simulink model "Lab3_1"  (R2021b)
settings: Solver=VariableStepAuto  StartTime=0.0  StopTime=10.0  RelTol=1e-3
libraries: fl_lib x7, nesl_utility x7, ee_lib x6, eeRmsMeasurement x5
settings Model: Creator=coolk  LastModifiedBy=coolk

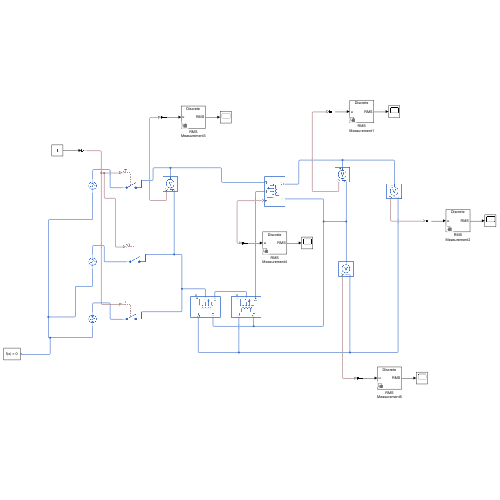
[thumbnail: Simulink's stored preview of the top-level diagram]
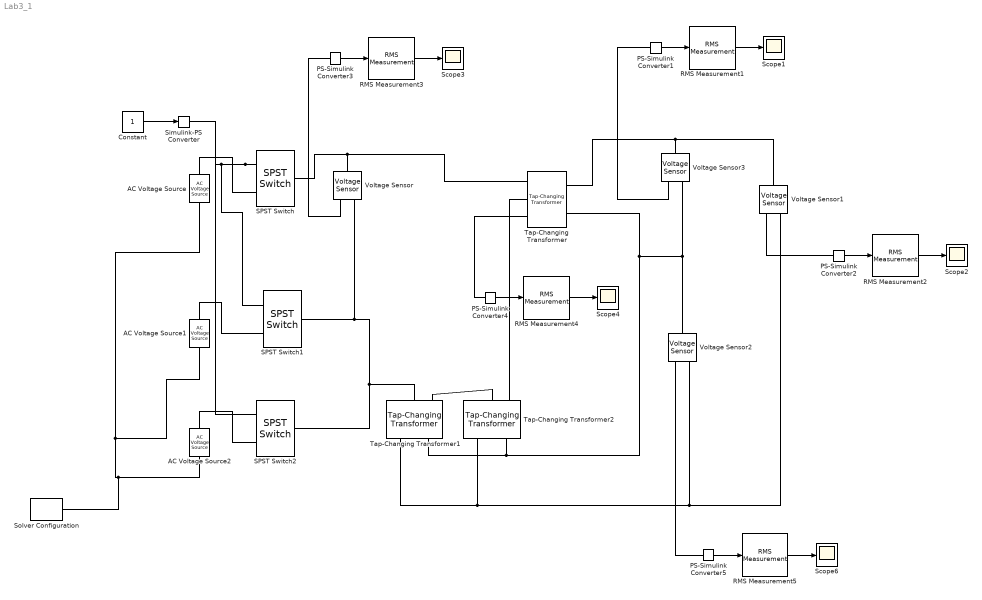
== system Lab3_1 ==
  AC Voltage Source : fl_lib/Electrical/Electrical Sources/AC Voltage Source  amp=1 V  shift=0 deg  frequency=60 Hz  omega=0 rad/s
  AC Voltage Source1 : fl_lib/Electrical/Electrical Sources/AC Voltage Source  amp=1 V  shift=0 deg  frequency=60 Hz  omega=0 rad/s
  AC Voltage Source2 : fl_lib/Electrical/Electrical Sources/AC Voltage Source  amp=1 V  shift=0 deg  frequency=60 Hz  omega=0 rad/s
  Constant : Constant
  PS-Simulink Converter{1..5} (5 alike) : nesl_utility/PS-Simulink Converter  PhysicalDomain=network_engine_domain  SubClassName=ps_output  LeftPortType=input  RightPortType=output  PseudoPeriodic=off  Frequencies=[]  Unit=inherit  AffineConversion=off
  RMS Measurement{1..5} (5 alike) : eeRmsMeasurement/RMS Measurement  LabelModeActiveChoice=Total  F=60  SpecifyHarmonics=off  K=[0 1 2]  Ts=10e-4
      settings: SourceProductBaseCode=PS
  SPST Switch : ee_lib/Switches & Breakers/SPST Switch  R_closed=0.01 Ohm  G_open=1e-6 S  Threshold=0.5 V  Width=0 V  model_dynamics=0  t_on=1e-3 s  t_off=1e-3 s  initial_vT=0 V
      settings: SourceProductBaseCode=PS  InternalSimscapePortConfiguration="{\"Bottom\":[],\"Left\":[{\"id\":\"vT\",\"label\":\"vT\",\"type\":\"input\"},{\"id\":\"p\",\"label\":\"\",\"type\":\"foundation.electrical.electrical\"}],\"Right\":[{\"id\":\"n\",\"label\":\"\",\"type\":\"foundation.electrical.electrical\"}],\"Top\":[]}"
  SPST Switch1 : ee_lib/Switches & Breakers/SPST Switch  R_closed=0.01 Ohm  G_open=1e-6 S  Threshold=0.5 V  Width=0 V  model_dynamics=0  t_on=1e-3 s  t_off=1e-3 s  initial_vT=0 V
      settings: SourceProductBaseCode=PS  InternalSimscapePortConfiguration="{\"Bottom\":[],\"Left\":[{\"id\":\"vT\",\"label\":\"vT\",\"type\":\"input\"},{\"id\":\"p\",\"label\":\"\",\"type\":\"foundation.electrical.electrical\"}],\"Right\":[{\"id\":\"n\",\"label\":\"\",\"type\":\"foundation.electrical.electrical\"}],\"Top\":[]}"
  SPST Switch2 : ee_lib/Switches & Breakers/SPST Switch  R_closed=0.01 Ohm  G_open=1e-6 S  Threshold=0.5 V  Width=0 V  model_dynamics=0  t_on=1e-3 s  t_off=1e-3 s  initial_vT=0 V
      settings: SourceProductBaseCode=PS  InternalSimscapePortConfiguration="{\"Bottom\":[],\"Left\":[{\"id\":\"vT\",\"label\":\"vT\",\"type\":\"input\"},{\"id\":\"p\",\"label\":\"\",\"type\":\"foundation.electrical.electrical\"}],\"Right\":[{\"id\":\"n\",\"label\":\"\",\"type\":\"foundation.electrical.electrical\"}],\"Top\":[]}"
  Scope{1..4,6} (5 alike) : Scope
  Simulink-PS Converter : nesl_utility/Simulink-PS Converter  PhysicalDomain=network_engine_domain  SubClassName=ps_input  LeftPortType=input  RightPortType=output  PseudoPeriodic=off  Frequencies=[]  NoiseDistribution=none  NoiseParameters=[]  Unit=1  AffineConversion=off  FilteringAndDerivatives=provide  SimscapeFilterOrder=1  InputFilterTimeConstant=0.001  UdotUserProvided=0
      settings: SourceProductBaseCode=PW,SS
  Solver Configuration : nesl_utility/Solver Configuration  PhysicalDomain=network_engine_domain  SubClassName=solver  LeftPortType=input  RightPortType=generic  Tones=[]  Harmonics=[]  SimulateNoise=off  Profile=off  UseLocalSampling=off  EnableSwitchedLinearOptims=on  FrequencyDomain=off  UseCCode=off  RelTol=0.001  AbsTol=1e-06  MinStep=1e-09  ToWorkspace=off  RevertToSquareIcSolve=off  NumHomotopyIterations=100  PhasorMode=off  PhasorModeNumHarmonics=1  DoDC=off  ResidualTolerance=1e-09  UseLocalSolver=off  LocalSolverChoice=NE_BACKWARD_EULER_ADVANCER  LocalSolverSampleTime=0.001  DoFixedCost=off  MaxNonlinIter=3  MaxModeIter=2  ComputeImpulses=off  ImpulseIterations=2  LinearAlgebra=auto  EquationFormulation=NE_TIME_EF  DelaysMemoryBudget=1024  AutomaticFiltering=on  FilteringTimeConstant=0.001  PartitionStorageMethod=AS_NEEDED  PartitionMemoryBudget=1024  PartitionMethod=ROBUST
      settings: SourceProductBaseCode=PW,SS
  Tap-Changing Transformer : ee_lib/Passive/Transformers/Tap-Changing Transformer  n0=1  Lp=1e-6 H  Ls=1e-6 H  Rm=1e6 Ohm  Lm=100e-6 H  Rp=0 Ohm  Rs=0 Ohm  Gp=0 1/Ohm  Gs=0 1/Ohm  prm=1  pmin=-5  pmax=5  delta=86.6  controlThreshold=0.5  i1_specify=off  i1_priority=None  i1=0 A  i1_nominal_specify=off  i1_nominal_unit=A  i1_nominal_value=1  i2_specify=off  i2_priority=None  i2=0 A  i2_nominal_specify=off  i2_nominal_unit=A  i2_nominal_value=1  tapPosition_specify=off  tapPosition_priority=High  tapPosition=0
      settings: SourceProductBaseCode=PS  InternalSimscapePortConfiguration="{\"Bottom\":[],\"Left\":[{\"id\":\"p1\",\"label\":\"1+\",\"type\":\"foundation.electrical.electrical\"},{\"id\":\"n1\",\"label\":\"1-\",\"type\":\"foundation.electrical.electrical\"},{\"id\":\"control\",\"label\":\"c\",\"type\":\"input\"}],\"Right\":[{\"id\":\"p2\",\"label\":\"2+\",\"type\":\"foundation.electrical.electrical\"},{\"id\":\"n2\",\"label\":\"2-\",\"type\":\"foundation.electrical.electrical\"}],\"Top\":[]}"
  Tap-Changing Transformer1 : ee_lib/Passive/Transformers/Tap-Changing Transformer  n0=1  Lp=1e-6 H  Ls=1e-6 H  Rm=1e6 Ohm  Lm=100e-6 H  Rp=0 Ohm  Rs=0 Ohm  Gp=0 1/Ohm  Gs=0 1/Ohm  prm=1  pmin=-5  pmax=5  delta=86.6  controlThreshold=0.5  i1_specify=off  i1_priority=None  i1=0 A  i1_nominal_specify=off  i1_nominal_unit=A  i1_nominal_value=1  i2_specify=off  i2_priority=None  i2=0 A  i2_nominal_specify=off  i2_nominal_unit=A  i2_nominal_value=1  tapPosition_specify=off  tapPosition_priority=High  tapPosition=0
      settings: SourceProductBaseCode=PS  InternalSimscapePortConfiguration="{\"Bottom\":[],\"Left\":[{\"id\":\"p1\",\"label\":\"1+\",\"type\":\"foundation.electrical.electrical\"},{\"id\":\"n1\",\"label\":\"1-\",\"type\":\"foundation.electrical.electrical\"},{\"id\":\"control\",\"label\":\"c\",\"type\":\"input\"}],\"Right\":[{\"id\":\"p2\",\"label\":\"2+\",\"type\":\"foundation.electrical.electrical\"},{\"id\":\"n2\",\"label\":\"2-\",\"type\":\"foundation.electrical.electrical\"}],\"Top\":[]}"
  Tap-Changing Transformer2 : ee_lib/Passive/Transformers/Tap-Changing Transformer  n0=1  Lp=1e-6 H  Ls=1e-6 H  Rm=1e6 Ohm  Lm=100e-6 H  Rp=0 Ohm  Rs=0 Ohm  Gp=0 1/Ohm  Gs=0 1/Ohm  prm=1  pmin=-5  pmax=5  delta=86.6  controlThreshold=0.5  i1_specify=off  i1_priority=None  i1=0 A  i1_nominal_specify=off  i1_nominal_unit=A  i1_nominal_value=1  i2_specify=off  i2_priority=None  i2=0 A  i2_nominal_specify=off  i2_nominal_unit=A  i2_nominal_value=1  tapPosition_specify=off  tapPosition_priority=High  tapPosition=0
      settings: SourceProductBaseCode=PS  InternalSimscapePortConfiguration="{\"Bottom\":[],\"Left\":[{\"id\":\"p1\",\"label\":\"1+\",\"type\":\"foundation.electrical.electrical\"},{\"id\":\"n1\",\"label\":\"1-\",\"type\":\"foundation.electrical.electrical\"},{\"id\":\"control\",\"label\":\"c\",\"type\":\"input\"}],\"Right\":[{\"id\":\"p2\",\"label\":\"2+\",\"type\":\"foundation.electrical.electrical\"},{\"id\":\"n2\",\"label\":\"2-\",\"type\":\"foundation.electrical.electrical\"}],\"Top\":[]}"
  Voltage Sensor{,1..3} (4 alike) : fl_lib/Electrical/Electrical Sensors/Voltage Sensor
  wires:
  Constant/1 -> Simulink-PS Converter/1
  RMS Measurement5/1 -> Scope6/1
  PS-Simulink Converter5/1 -> RMS Measurement5/1
  RMS Measurement1/1 -> Scope1/1
  PS-Simulink Converter1/1 -> RMS Measurement1/1
  RMS Measurement2/1 -> Scope2/1
  PS-Simulink Converter2/1 -> RMS Measurement2/1
  RMS Measurement3/1 -> Scope3/1
  PS-Simulink Converter3/1 -> RMS Measurement3/1
  RMS Measurement4/1 -> Scope4/1
  PS-Simulink Converter4/1 -> RMS Measurement4/1
  connections:
  SPST Switch/LConn1 -- SPST Switch1/LConn1 -- Simulink-PS Converter/RConn1 -- SPST Switch2/LConn1
  AC Voltage Source/RConn1 -- AC Voltage Source1/RConn1 -- Solver Configuration/RConn1 -- AC Voltage Source2/RConn1
  AC Voltage Source1/LConn1 -- SPST Switch1/LConn2
  AC Voltage Source/LConn1 -- SPST Switch/LConn2
  AC Voltage Source2/LConn1 -- SPST Switch2/LConn2
  Voltage Sensor/RConn2 -- SPST Switch2/RConn1 -- Tap-Changing Transformer1/LConn2 -- SPST Switch1/RConn1
  Voltage Sensor3/RConn2 -- Voltage Sensor2/LConn1 -- Tap-Changing Transformer1/RConn1 -- Tap-Changing Transformer2/RConn1 -- Tap-Changing Transformer/RConn2
  Voltage Sensor3/LConn1 -- Tap-Changing Transformer/RConn1 -- Voltage Sensor1/LConn1
  Voltage Sensor2/RConn2 -- Tap-Changing Transformer2/RConn2 -- Tap-Changing Transformer1/RConn2 -- Voltage Sensor1/RConn2
  Voltage Sensor2/RConn1 -- PS-Simulink Converter5/LConn1
  Voltage Sensor3/RConn1 -- PS-Simulink Converter1/LConn1
  Voltage Sensor1/RConn1 -- PS-Simulink Converter2/LConn1
  Voltage Sensor/RConn1 -- PS-Simulink Converter3/LConn1
  SPST Switch/RConn1 -- Tap-Changing Transformer/LConn1 -- Voltage Sensor/LConn1
  Tap-Changing Transformer/LConn3 -- PS-Simulink Converter4/LConn1
  Tap-Changing Transformer/LConn2 -- Tap-Changing Transformer2/LConn1
  Tap-Changing Transformer2/LConn2 -- Tap-Changing Transformer1/LConn1
